simulink model "simuNoLinearControl"  (R2021a)
settings: Solver=VariableStepAuto  StartTime=0.0  StopTime=2000  MaxStep=0.01  RelTol=1e-3
values from neighbouring files (symbols this model uses):
  a = 0.86    [ProjetoControleTanqueConicoFinal.m]    (also in TrabalhoTanqueConico.m = 4*A2*sqrt(2*g)/(pi*0.6^2); TrabalhoTanqueConicoOutraVersao.m = 4*A2*sqrt(2*g)/(pi*0.6^2))
  b = 3.53    [ProjetoControleTanqueConicoFinal.m]    (also in TrabalhoTanqueConico.m = 3.53677651315; TrabalhoTanqueConicoOutraVersao.m = 3.53677651315)
  d = 0.6    [ProjetoControleTanqueConicoFinal.m]
  hbar = 6    [ProjetoControleTanqueConicoFinal.m]    (also in TrabalhoTanqueConico.m = 5; TrabalhoTanqueConicoOutraVersao.m = 5)
  k1 = K(1,1)    [ProjetoControleTanqueConicoFinal.m]
  k2 = K(1,2)    [ProjetoControleTanqueConicoFinal.m]
  x1ini = 0.05    [ProjetoControleTanqueConicoFinal.m]
  x2ini = -0.5    [ProjetoControleTanqueConicoFinal.m]
settings Model: Creator=danie  LastModifiedBy=guilh
settings SolverCC: AlgebraicLoopSolver=TrustRegion
settings DataIOCC: ReturnWorkspaceOutputs=off
settings DebuggingCC: SFMachineParentedDataDiag=warning  ArithmeticOperatorsInVariantConditions=warning
settings SFSimCC: SimUseLocalCustomCode=off  CustomCodeUndefinedFunction=UseInterfaceOnly
settings RTWCC: RTWUseLocalCustomCode=off

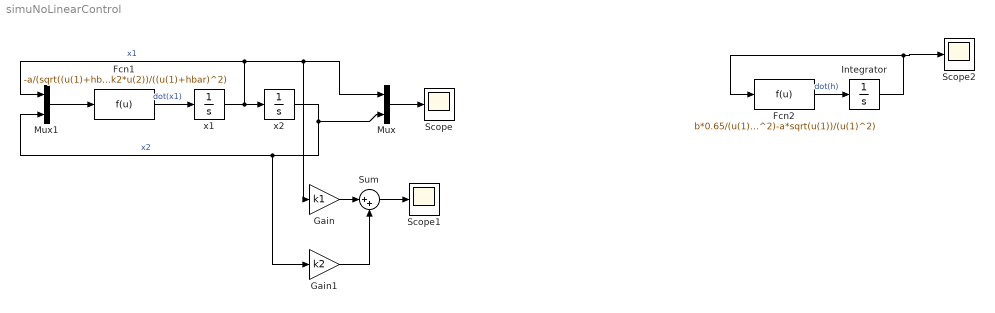
== system simuNoLinearControl ==
  Fcn1 : Fcn  Expr=-a/(sqrt((u(1)+hbar)^3)) + b*d/((u(1)+hbar)^2)+b*(k1*u(1)+k2*u(2))/((u(1)+hbar)^2)
  Fcn2 : Fcn  Expr=b*0.65/(u(1)^2)-a*sqrt(u(1))/(u(1)^2)
  Gain : Gain  Gain=k1
  Gain1 : Gain  Gain=k2
  Integrator : Integrator  InitialCondition=6
  Mux : Mux  Inputs=2
  Mux1 : Mux  Inputs=2
  Scope : Scope
  Scope1 : Scope
  Scope2 : Scope
  Sum : Sum  Inputs=|++
  x1 : Integrator  InitialCondition=x1ini
  x2 : Integrator  InitialCondition=x2ini
  wires:
  x1/1 -> Mux1/1, Gain/1, Mux/1, x2/1  "x1"
  Fcn1/1 -> x1/1  "dot(x1)"
  Mux1/1 -> Fcn1/1
  x2/1 -> Mux/2, Gain1/1, Mux1/2  "x2"
  Mux/1 -> Scope/1
  Gain/1 -> Sum/1
  Gain1/1 -> Sum/2
  Sum/1 -> Scope1/1
  Fcn2/1 -> Integrator/1  "dot(h)"
  Integrator/1 -> Fcn2/1, Scope2/1
